simulink model "PID"  (R2018b)
settings: Solver=ode4  StartTime=0.0  StopTime=100  FixedStep=0.002  RelTol=1e-3
undefined symbols (not defined in the file): delta_negative_l, delta_negative_r, delta_positive_l, delta_positive_r, K_l, K_r, kd_l, kd_r, ki_l, ki_r, kp_l, kp_r, tau_l, tau_r
settings Model: Creator=pedro  LastModifiedBy=Pedro Saman
settings SFSimCC: SimUseLocalCustomCode=off
settings RTWCC: RTWUseLocalCustomCode=off
settings CodeAppCC: StateflowObjectComments=on

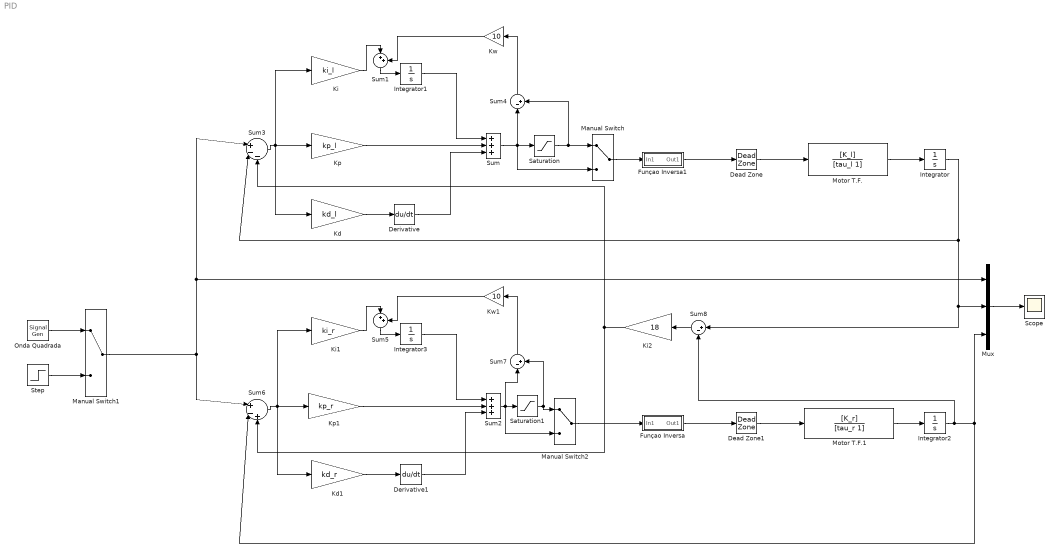
== system PID ==
  Dead Zone : DeadZone  LowerValue=delta_negative_l  UpperValue=delta_positive_l  SaturateOnIntegerOverflow=on
  Dead Zone1 : DeadZone  LowerValue=delta_negative_r  UpperValue=delta_positive_r  SaturateOnIntegerOverflow=on
  Derivative : Derivative
  Derivative1 : Derivative
  Funçao Inversa : Subsystem
  Funçao Inversa1 : Subsystem
  Integrator{,1..3} (4 alike) : Integrator
  Kd : Gain  Gain=kd_l
  Kd1 : Gain  Gain=kd_r
  Ki : Gain  Gain=ki_l
  Ki1 : Gain  Gain=ki_r
  Ki2 : Gain  Gain=18
  Kp : Gain  Gain=kp_l
  Kp1 : Gain  Gain=kp_r
  Kw : Gain  Gain=10
  Kw1 : Gain  Gain=10
  Manual Switch : ManualSwitch
  Manual Switch1 : ManualSwitch
  Manual Switch2 : ManualSwitch
  Motor T.F. : TransferFcn  Numerator=[K_l]  Denominator=[tau_l 1]
  Motor T.F.1 : TransferFcn  Numerator=[K_r]  Denominator=[tau_r 1]
  Mux : Mux  Inputs=3
  Onda Quadrada : SignalGenerator  WaveForm=square  Amplitude=5600  Units=rad/sec
  Saturation : Saturate  UpperLimit=14.4  LowerLimit=-14.4
  Saturation1 : Saturate  UpperLimit=14.4  LowerLimit=-14.4
  Scope : Scope
  Step : Step  After=100  SampleTime=0
  Sum : Sum  Inputs=|+|+|+|
  Sum1 : Sum  Inputs=|++
  Sum2 : Sum  Inputs=|+|+|+|
  Sum3 : Sum  Inputs=|+--
  Sum4 : Sum  Inputs=|-+
  Sum5 : Sum  Inputs=|++
  Sum6 : Sum  Inputs=|+-+
  Sum7 : Sum  Inputs=|-+
  Sum8 : Sum  Inputs=|+-
  wires:
  Motor T.F./1 -> Integrator/1
  Dead Zone/1 -> Motor T.F./1
  Integrator/1 -> Sum8/1, Mux/2, Sum3/2
  Kd/1 -> Derivative/1
  Integrator1/1 -> Sum/1
  Sum/1 -> Saturation/1, Manual Switch/2, Sum4/1
  Saturation/1 -> Manual Switch/1, Sum4/2
  Sum4/1 -> Kw/1
  Ki/1 -> Sum1/1
  Sum1/1 -> Integrator1/1
  Kw/1 -> Sum1/2
  Funçao Inversa1/1(Out1) -> Dead Zone/1
  Manual Switch1/1 -> Sum6/1, Mux/1, Sum3/1
  Derivative/1 -> Sum/3
  Motor T.F.1/1 -> Integrator2/1
  Dead Zone1/1 -> Motor T.F.1/1
  Funçao Inversa/1(Out1) -> Dead Zone1/1
  Sum7/1 -> Kw1/1
  Kd1/1 -> Derivative1/1
  Saturation1/1 -> Sum7/2, Manual Switch2/1
  Kw1/1 -> Sum5/2
  Ki1/1 -> Sum5/1
  Derivative1/1 -> Sum2/3
  Sum2/1 -> Sum7/1, Manual Switch2/2, Saturation1/1
  Integrator3/1 -> Sum2/1
  Sum5/1 -> Integrator3/1
  Step/1 -> Manual Switch1/2
  Onda Quadrada/1 -> Manual Switch1/1
  Mux/1 -> Scope/1
  Integrator2/1 -> Sum6/2, Mux/3, Sum8/2
  Sum3/1 -> Ki/1, Kd/1, Kp/1
  Sum6/1 -> Kd1/1, Ki1/1, Kp1/1
  Kp/1 -> Sum/2
  Manual Switch/1 -> Funçao Inversa1/1(In1)
  Manual Switch2/1 -> Funçao Inversa/1(In1)
  Kp1/1 -> Sum2/2
  Sum8/1 -> Ki2/1
  Ki2/1 -> Sum6/3, Sum3/3

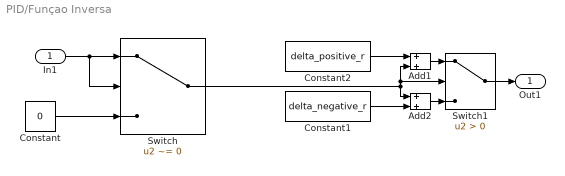
== system PID/Funçao Inversa ==
  In1 : Inport
  Add1 : Sum
  Add2 : Sum
  Constant : Constant  Value=0
  Constant1 : Constant  Value=delta_negative_r
  Constant2 : Constant  Value=delta_positive_r
  Switch : Switch  Criteria=u2 ~= 0
  Switch1 : Switch  Criteria=u2 > Threshold
  Out1 : Outport
  wires:
  Switch/1 -> Add1/2, Switch1/2, Add2/1
  Constant1/1 -> Add2/2
  In1/1 -> Switch/2, Switch/1
  Constant/1 -> Switch/3
  Switch1/1 -> Out1/1
  Add2/1 -> Switch1/3
  Add1/1 -> Switch1/1
  Constant2/1 -> Add1/1

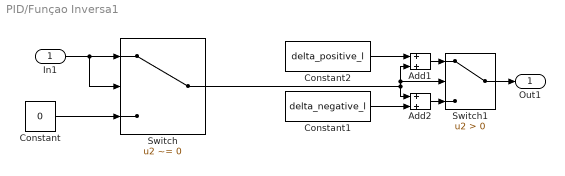
== system PID/Funçao Inversa1 ==
  In1 : Inport
  Add1 : Sum
  Add2 : Sum
  Constant : Constant  Value=0
  Constant1 : Constant  Value=delta_negative_l
  Constant2 : Constant  Value=delta_positive_l
  Switch : Switch  Criteria=u2 ~= 0
  Switch1 : Switch  Criteria=u2 > Threshold
  Out1 : Outport
  wires:
  Switch/1 -> Add1/2, Switch1/2, Add2/1
  Constant1/1 -> Add2/2
  In1/1 -> Switch/2, Switch/1
  Constant/1 -> Switch/3
  Switch1/1 -> Out1/1
  Add2/1 -> Switch1/3
  Add1/1 -> Switch1/1
  Constant2/1 -> Add1/1
